simulink model "BifurcationODE"  (R2022a)
settings: Solver=VariableStepAuto  StartTime=0.0  StopTime=10.0  RelTol=1e-3
undefined symbols (not defined in the file): a, R, Rc
settings Model: Creator=Adam Ghatta  LastModifiedBy=Adam Ghatta

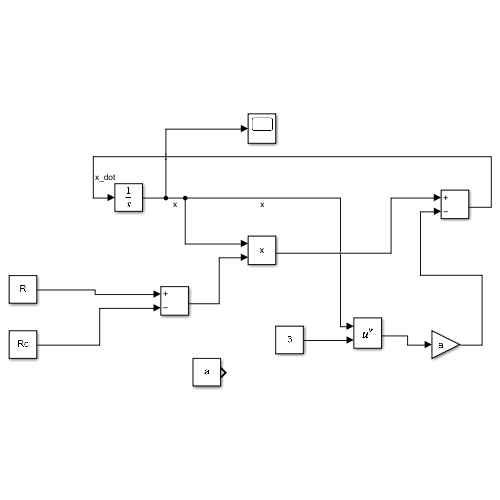
[thumbnail: Simulink's stored preview of the top-level diagram]
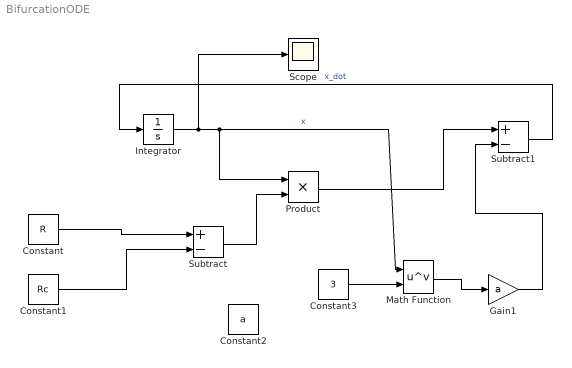
== system BifurcationODE ==
  Constant : Constant  Value=R
  Constant1 : Constant  Value=Rc
  Constant2 : Constant  Value=a
  Constant3 : Constant  Value=3
  Gain1 : Gain  Gain=a
  Integrator : Integrator  InitialCondition=.2
  Math Function : Math  Operator=pow  OutputSignalType=real
  Product : Product
  Scope : Scope
  Subtract : Sum  Inputs=+-
  Subtract1 : Sum  Inputs=+-
  wires:
  Integrator/1 -> Scope/1, Math Function/1, Product/1  "x"
  Subtract1/1 -> Integrator/1  "x_dot"
  Constant/1 -> Subtract/1
  Constant1/1 -> Subtract/2
  Subtract/1 -> Product/2
  Constant3/1 -> Math Function/2
  Math Function/1 -> Gain1/1
  Product/1 -> Subtract1/1
  Gain1/1 -> Subtract1/2
